simulink model "OFDM_project"  (R2018a)
settings: Solver=VariableStepAuto  StartTime=0.0  StopTime=0.1  RelTol=1e-3
undefined symbols (not defined in the file or in its folder): doppler
libraries: commchan3 x3, commofdm x3, commdigbbndam3 x3, commsink2 x2, commrandsrc3 x1, dspstat3 x1
settings Model: Creator=Areeb  LastModifiedBy=Areeb

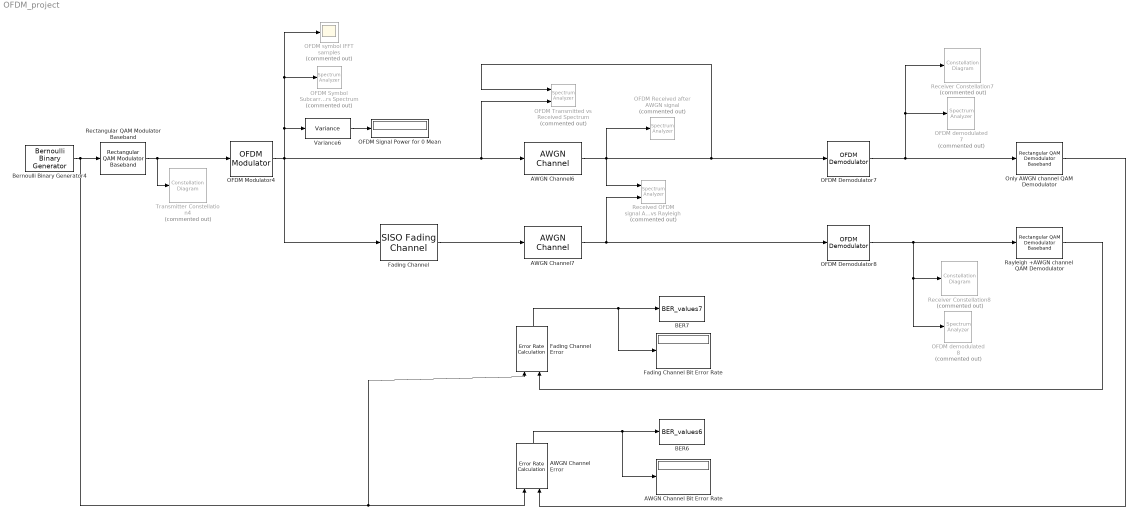
== system OFDM_project ==
  AWGN Channel6 : commchan3/AWGN Channel  InputProcessing=Columns as channels (frame based)  seed=67  noiseMode="Signal to noise ratio  (Eb/No)"  EbNodB=10  EsNodB=10  SNRdB=10  bitsPerSym=192  Ps=0.029  Tsym=4e-6  variance=1
  AWGN Channel7 : commchan3/AWGN Channel  InputProcessing=Columns as channels (frame based)  seed=67  noiseMode="Signal to noise ratio  (Eb/No)"  EbNodB=10  EsNodB=10  SNRdB=10  bitsPerSym=192  Ps=0.029  Tsym=4e-6  variance=1
  AWGN Channel Bit Error Rate : Display
  AWGN Channel Error : commsink2/Error Rate Calculation  N=0  st_delay=0  cp_mode=Entire frame  subframe=[]  PMode=Port  WsName=ErrorVec  RsMode2=off  stop=off  numErr=100  maxBits=1e6
  BER6 : ToWorkspace  VariableName=BER_values6  SampleTime=-1
      settings: Save2DSignal=2-D array (concatenate along first dimension)
  BER7 : ToWorkspace  VariableName=BER_values7  SampleTime=-1
      settings: Save2DSignal=2-D array (concatenate along first dimension)
  Bernoulli Binary Generator4 : commrandsrc3/Bernoulli Binary Generator  ProbabilityOfZero=0.5  SeedSource=Auto  Seed=0  SampleTime=1/20e6  SamplesPerFrame=192  OutputDataType=double  SimulateUsing=Interpreted execution
  Fading Channel : commchan3/SISO Fading Channel  InheritSampleRate=on  SampleRate=312.5e3  PathDelays=[0 1e-9]  AveragePathGains=[0 -3]  NormalizePathGains=on  FadingDistribution=Rayleigh  KFactor=3  DirectPathDopplerShift=0  DirectPathInitialPhase=0  MaximumDopplerShift=0  DopplerSpectrum=doppler('Jakes')  ChannelInterpolationMethod=Polyphase  RandomStream=mt19937ar with seed  RandomNumGenerator=mt19937ar  Seed=73  PathGainsOutputPort=off  ChannelFilterDelayOutputPort=off  SimulateUsing=Interpreted execution  Visualization=Off  PathsForDopplerDisplay=1  SamplesToDisplay=100%
      settings: SourceProductName=Communications System Toolbox
  Fading Channel Bit Error Rate : Display
  Fading Channel Error : commsink2/Error Rate Calculation  N=0  st_delay=0  cp_mode=Entire frame  subframe=[]  PMode=Port  WsName=ErrorVec  RsMode2=off  stop=off  numErr=100  maxBits=1e6
  OFDM Demodulator7 : commofdm/OFDM Demodulator  FFTLength=64  NumGuardBandCarriers=[8; 7]  RemoveDCCarrier=on  PilotOutputPort=off  PilotCarrierIndices=[12; 26; 40; 50]  CyclicPrefixLength=16  NumSymbols=1  NumReceiveAntennas=1  SimulateUsing=Interpreted execution
      settings: SourceProductName=Communications System Toolbox  SourceProductBaseCode=CM
  OFDM Demodulator8 : commofdm/OFDM Demodulator  FFTLength=64  NumGuardBandCarriers=[8; 7]  RemoveDCCarrier=on  PilotOutputPort=off  PilotCarrierIndices=[12; 26; 40; 50]  CyclicPrefixLength=16  NumSymbols=1  NumReceiveAntennas=1  SimulateUsing=Interpreted execution
      settings: SourceProductName=Communications System Toolbox  SourceProductBaseCode=CM
  OFDM Modulator4 : commofdm/OFDM Modulator  FFTLength=64  NumGuardBandCarriers=[8; 7]  InsertDCNull=on  PilotInputPort=off  PilotCarrierIndices=[12; 26; 40; 50]  CyclicPrefixLength=16  Windowing=off  WindowLength=1  NumSymbols=1  NumTransmitAntennas=1  SimulateUsing=Interpreted execution
      settings: SourceProductName=Communications System Toolbox  SourceProductBaseCode=CM
  OFDM Received after AWGN signal : SpectrumAnalyzer  Commented=on
  OFDM Signal Power for 0 Mean : Display
  OFDM Symbol Subcarriers Spectrum : SpectrumAnalyzer  Commented=on
  OFDM Transmitted vs Received Spectrum : SpectrumAnalyzer  Commented=on  NumInputPorts=2
  OFDM demodulated 7 : SpectrumAnalyzer  Commented=on
  OFDM demodulated 8 : SpectrumAnalyzer  Commented=on
  OFDM symbol IFFT samples : Scope  Commented=on
  Only AWGN channel QAM Demodulator : commdigbbndam3/Rectangular QAM Demodulator Baseband  M=16  OutType=Bit  DecType=Hard decision  VarSource=Dialog  Variance=1  Dec=Gray  Mapping=[0:15]  PowType=Min. distance between symbols  MinDist=1  AvgPow=0.2  PeakPow=1  Ph=0  outDtype1=Inherit via internal rule  outDtype2=Inherit via internal rule  derotateFactorWordLen=16  derotateFactorDataTypeStr=Inherit: Same word length as input  derotateFactorLastDataTypeStr=Inherit: Same word length as input  denormFactorWordLen=16  denormFactorDataTypeStr=Inherit: Same word length as input  denormFactorLastDataTypeStr=Inherit: Same word length as input  prodOutWordLen=32  prodOutOverflowMode=Wrap  prodOutRoundingMode=Floor  prodOutOvFlMode=off  prodOutOvFlModeLastStrValue=off  sumWordLen=32
  Rayleigh +AWGN channel QAM Demodulator : commdigbbndam3/Rectangular QAM Demodulator Baseband  M=16  OutType=Bit  DecType=Hard decision  VarSource=Dialog  Variance=1  Dec=Gray  Mapping=[0:15]  PowType=Min. distance between symbols  MinDist=1  AvgPow=1  PeakPow=1  Ph=0  outDtype1=Inherit via internal rule  outDtype2=Inherit via internal rule  derotateFactorWordLen=16  derotateFactorDataTypeStr=Inherit: Same word length as input  derotateFactorLastDataTypeStr=Inherit: Same word length as input  denormFactorWordLen=16  denormFactorDataTypeStr=Inherit: Same word length as input  denormFactorLastDataTypeStr=Inherit: Same word length as input  prodOutWordLen=32  prodOutOverflowMode=Wrap  prodOutRoundingMode=Floor  prodOutOvFlMode=off  prodOutOvFlModeLastStrValue=off  sumWordLen=32
  Received OFDM signal AWGN vs Rayleigh : SpectrumAnalyzer  Commented=on  NumInputPorts=2
  Receiver Constellation7 : ConstellationDiagram  Commented=on
  Receiver Constellation8 : ConstellationDiagram  Commented=on
  Rectangular QAM Modulator Baseband : commdigbbndam3/Rectangular QAM Modulator Baseband  M=16  InType=Bit  Enc=Gray  Mapping=[0:15]  PowType=Min. distance between symbols  MinDist=1  AvgPow=0.2  PeakPow=1  Ph=0  outDtype=double  outWordLen=16  outUDDataType=sfix(16)  outFracLenMode=Best precision  outFracLen=15  outDataTypeStr=double  outLastDataTypeStr=double
  Transmitter Constellation4 : ConstellationDiagram  Commented=on
  Variance6 : dspstat3/Variance  run=off  InputProcessing=Columns as channels (frame based)  reset_popup=None  directionMode=Each column  dimension=1  roiEnable=off  roiType=Rectangles  roiPortion=Entire ROI  roiOutput=Individual statistics for each ROI  roiFlag=off  roundingMode=Floor  overflowMode=off
      settings: SourceProductName=DSP System Toolbox
  wires:
  AWGN Channel7/1 -> Received OFDM signal AWGN vs Rayleigh/2, OFDM Demodulator8/1
  Only AWGN channel QAM Demodulator/1 -> AWGN Channel Error/2
  Rayleigh +AWGN channel QAM Demodulator/1 -> Fading Channel Error/2
  Fading Channel Error/1 -> Fading Channel Bit Error Rate/1, BER7/1
  Rectangular QAM Modulator Baseband/1 -> OFDM Modulator4/1, Transmitter Constellation4/1
  OFDM Modulator4/1 -> Fading Channel/1, OFDM Transmitted vs Received Spectrum/2, AWGN Channel6/1, OFDM symbol IFFT samples/1, OFDM Symbol Subcarriers Spectrum/1, Variance6/1
  AWGN Channel6/1 -> Received OFDM signal AWGN vs Rayleigh/1, OFDM Transmitted vs Received Spectrum/1, OFDM Demodulator7/1, OFDM Received after AWGN signal/1
  OFDM Demodulator7/1 -> Only AWGN channel QAM Demodulator/1, Receiver Constellation7/1, OFDM demodulated 7/1
  Bernoulli Binary Generator4/1 -> Rectangular QAM Modulator Baseband/1, AWGN Channel Error/1, Fading Channel Error/1
  Fading Channel/1 -> AWGN Channel7/1
  Variance6/1 -> OFDM Signal Power for 0 Mean/1
  OFDM Demodulator8/1 -> Rayleigh +AWGN channel QAM Demodulator/1, OFDM demodulated 8/1, Receiver Constellation8/1
  AWGN Channel Error/1 -> BER6/1, AWGN Channel Bit Error Rate/1
